simulink model "hallsensor"  (R2013a)
settings: Solver=ode3  SolverMode=SingleTasking  StartTime=0.0  StopTime=inf  RelTol=1e-3
libraries: arduinolib x12
settings Model: SimulationMode=external  ExtModeTrigDuration=2  Creator=Sony  LastModifiedBy=Sony
settings OptimizationCC: OptimizeModelRefInitCode=on  LifeSpan=Inf
settings DebuggingCC: SolverPrmCheckMsg=none
settings HardwareCC: ProdBitPerInt=16  ProdBitPerPointer=8  ProdIntDivRoundTo=Zero  ProdEndianess=LittleEndian  ProdWordSize=8  ProdHWDeviceType=Atmel->AVR  TargetBitPerInt=16  TargetBitPerPointer=8  TargetIntDivRoundTo=Zero  TargetEndianess=LittleEndian  TargetWordSize=8  TargetHWDeviceType=Atmel->AVR
settings RTWCC: SystemTargetFile=realtime.tlc  GenerateMakefile=off  TemplateMakefile=realtime.tmf  Description=Run on Target Hardware  RTWVerbose=off  ProcessScript=realtime_make_rtw_hook
settings STFCustomTargetCC: TargetLibSuffix=.a  GenerateSampleERTMain=on  ERTCustomFileBanners=on  SupportNonInlinedSFcns=off  SupportVariableSizeSignals=on  MATLABClassNameForMDSCustomization=Simulink.SoftwareTarget.ERTCustomization  SystemTargetFile=realtime.tlc
settings ERTTargetCC: ParMdlRefBuildCompliant=off  CompOptLevelCompliant=off  ConcurrentExecutionCompliant=off  CombineOutputUpdateFcns=off  ERTFirstTimeCompliant=off  SupportContinuousTime=on  SupportVariableSizeSignals=on  ModelStepFunctionPrototypeControlCompliant=off  CPPClassGenCompliant=off  ExtModeTransport=3  ExtModeMexFile=ext_serial_win32_comm  ExtModeMexArgs=0 5 115200  ERTSrcFileBannerTemplate=realtime_code_template.cgt  ERTHdrFileBannerTemplate=realtime_code_template.cgt  ERTDataSrcFileTemplate=realtime_code_template.cgt  ERTDataHdrFileTemplate=realtime_code_template.cgt  ERTCustomFileTemplate=realtime_file_process.tlc

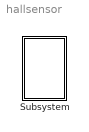
== system hallsensor ==
  Subsystem : Subsystem  mask{T=0.00001}

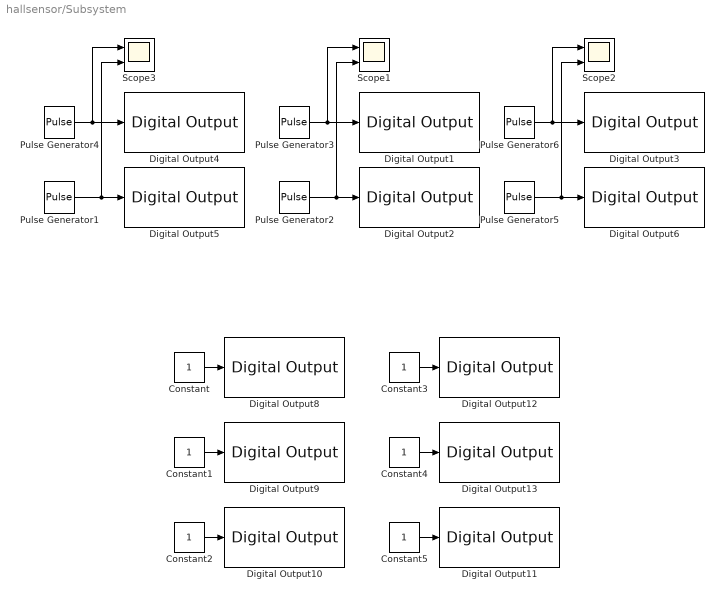
== system hallsensor/Subsystem ==
  Constant{,1..5} (6 alike) : Constant
  Digital Output1 : arduinolib/Digital Output  pinNumber=4
  Digital Output10 : arduinolib/Digital Output  pinNumber=12
  Digital Output11 : arduinolib/Digital Output  pinNumber=13
  Digital Output12 : arduinolib/Digital Output  pinNumber=9
  Digital Output13 : arduinolib/Digital Output  pinNumber=11
  Digital Output2 : arduinolib/Digital Output  pinNumber=5
  Digital Output3 : arduinolib/Digital Output  pinNumber=6
  Digital Output4 : arduinolib/Digital Output  pinNumber=2
  Digital Output5 : arduinolib/Digital Output  pinNumber=3
  Digital Output6 : arduinolib/Digital Output  pinNumber=7
  Digital Output8 : arduinolib/Digital Output  pinNumber=8
  Digital Output9 : arduinolib/Digital Output  pinNumber=10
  Pulse Generator1 : DiscretePulseGenerator  PulseType=Time based  Period=T  PulseWidth=50  PhaseDelay=T/2  SampleTime=0.002
  Pulse Generator2 : DiscretePulseGenerator  PulseType=Time based  Period=T  PulseWidth=50  PhaseDelay=T/3+T/2  SampleTime=0.002
  Pulse Generator3 : DiscretePulseGenerator  PulseType=Time based  Period=T  PulseWidth=50  PhaseDelay=T/3  SampleTime=0.002
  Pulse Generator4 : DiscretePulseGenerator  PulseType=Time based  Period=T  PulseWidth=50  SampleTime=0.002
  Pulse Generator5 : DiscretePulseGenerator  PulseType=Time based  Period=T  PulseWidth=50  PhaseDelay=T*(2/3)+T/2  SampleTime=0.002
  Pulse Generator6 : DiscretePulseGenerator  PulseType=Time based  Period=T  PulseWidth=50  PhaseDelay=T*(2/3)  SampleTime=0.002
  Scope1 : Scope  NumInputPorts=2
      settings: YMin=-5~-5  YMax=5~5
  Scope2 : Scope  NumInputPorts=2
      settings: YMin=-5~-5  YMax=5~5
  Scope3 : Scope  NumInputPorts=2
      settings: YMin=-5~-5  YMax=5~5  SaveName=ScopeData3
  wires:
  Constant/1 -> Digital Output8/1
  Constant4/1 -> Digital Output13/1
  Pulse Generator1/1 -> Scope3/2, Digital Output5/1
  Constant2/1 -> Digital Output10/1
  Constant3/1 -> Digital Output12/1
  Constant5/1 -> Digital Output11/1
  Constant1/1 -> Digital Output9/1
  Pulse Generator4/1 -> Scope3/1, Digital Output4/1
  Pulse Generator5/1 -> Scope2/2, Digital Output6/1
  Pulse Generator6/1 -> Scope2/1, Digital Output3/1
  Pulse Generator3/1 -> Scope1/1, Digital Output1/1
  Pulse Generator2/1 -> Scope1/2, Digital Output2/1
